simulink model "calculation_of_thrust"  (R2018b)
settings: Solver=FixedStepAuto  StartTime=0.0  StopTime=180  RelTol=1e-3
undefined symbols (not defined in the file): water, wr
settings Model: Creator=martin  LastModifiedBy=martin
settings DataIOCC: SaveOutput=off  SaveTime=off

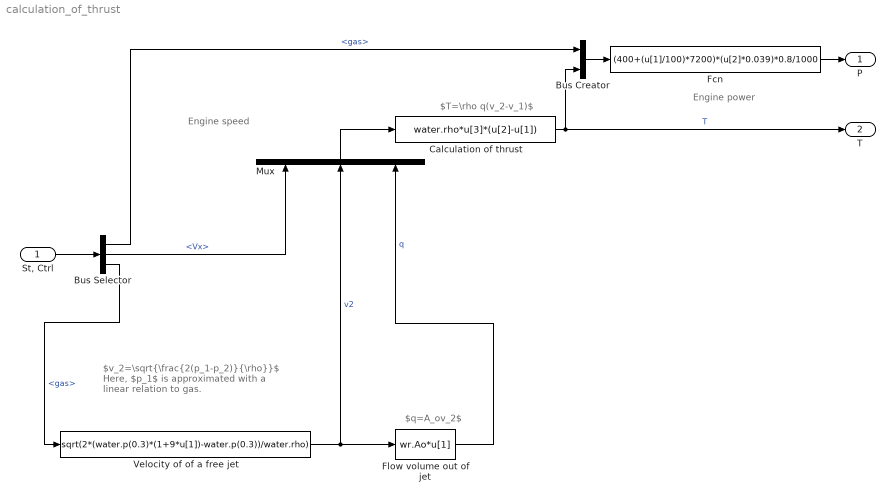
== system calculation_of_thrust ==
  note: Engine power
  note: Engine speed
  note: $v_2=\sqrt{\frac{2(p_1-p_2)}{\rho}}$
      | Here, $p_1$ is approximated with a linear
      | relation to gas.
  note: $T=\rho q(v_2-v_1)$
  note: $q=A_ov_2$
  "St, Ctrl" : Inport  OutDataTypeStr=Bus: slBus1
  Bus Creator : BusCreator  Inputs=2
  Bus Selector : BusSelector  OutputSignals=Control.gas,State.Vx,Control.gas
  Calculation of thrust : Fcn  Expr=water.rho*u[3]*(u[2]-u[1])
  Fcn : Fcn  Expr=(400+(u[1]/100)*7200)*(u[2]*0.039)*0.8/1000
  Flow volume out of jet : Fcn  Expr=wr.Ao*u[1]
  Mux : Mux  Inputs=3
  Velocity of of a free jet : Fcn  Expr=sqrt(2*(water.p(0.3)*(1+9*u[1])-water.p(0.3))/water.rho)
  P : Outport  OutDataTypeStr=double  PortDimensions=1  SampleTime=0
  T : Outport  Port=2
  wires:
  Calculation of thrust/1 -> Bus Creator/2, T/1  "T"
  Mux/1 -> Calculation of thrust/1
  Bus Selector/3 -> Velocity of of a free jet/1  "<gas>"
  Velocity of of a free jet/1 -> Mux/2, Flow volume out of jet/1  "v2"
  Flow volume out of jet/1 -> Mux/3  "q"
  Bus Selector/2 -> Mux/1  "<Vx>"
  "St, Ctrl"/1 -> Bus Selector/1
  Bus Selector/1 -> Bus Creator/1  "<gas>"
  Bus Creator/1 -> Fcn/1
  Fcn/1 -> P/1
